simulink model "lab4_5"  (R2022b)
settings: Solver=ode5  StartTime=0.0  StopTime=10.0  FixedStep=0.1  RelTol=1e-3
values from neighbouring files (symbols this model uses):
  A0 = A0*1.5-A0*A0'*A0*0.5    [lab4.m]
  I_rotor = 0    [lab4.m]
  J = [I_x 0 0 ; 0 I_y 0; 0 0 I_z]    [lab4.m]
  k_rotor = [0, 0, 1]    [lab4.m]
  M = [M_x M_y M_z]    [lab4.m]
  omega = [omega_x, omega_y, omega_z]    [lab4.m]
  omega_rotor = 0    [lab4.m]
  q = 0.5.*OMEGA*q    [lab4.m]
libraries: vrlib x2
settings Model: Creator=paole  LastModifiedBy=a1pab
settings SolverCC: AlgebraicLoopSolver=TrustRegion
settings DebuggingCC: UnconnectedInputMsg=warning  UnconnectedOutputMsg=warning  UnconnectedLineMsg=warning  SFMachineParentedDataDiag=warning
settings ModelReferenceCC: EnableRefExpFcnMdlSchedulingChecks=on
settings RTWCC: DLArmComputeVersion=19.05

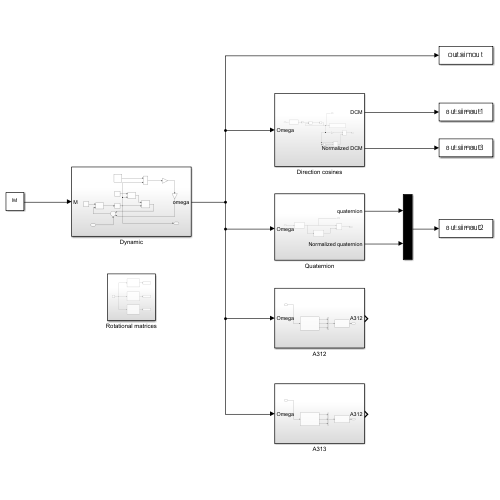
[thumbnail: Simulink's stored preview of the top-level diagram]
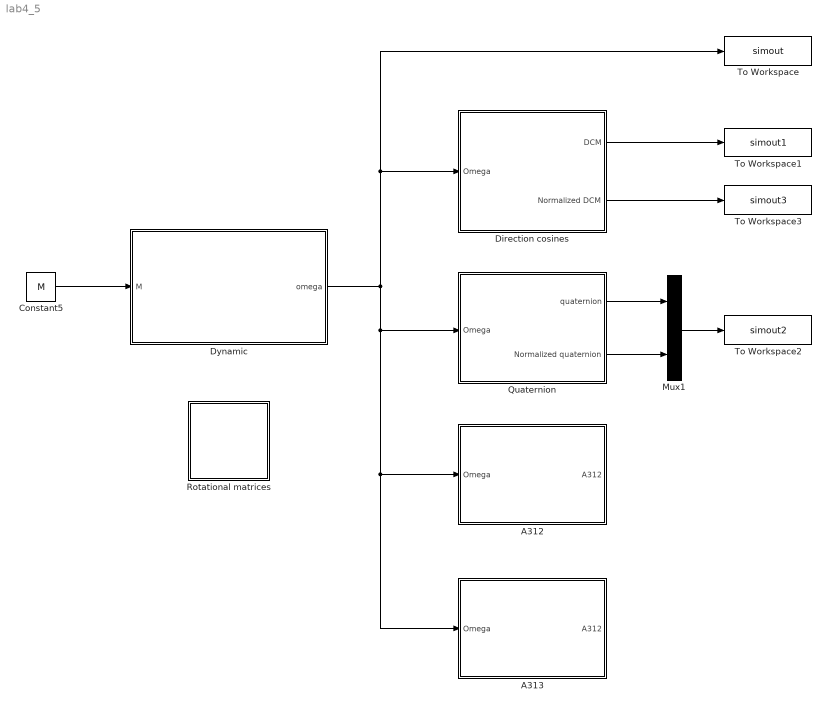
== system lab4_5 ==
  A312 : Subsystem
  A313 : Subsystem
  Constant5 : Constant  Value=M
  Direction cosines : Subsystem
  Dynamic : Subsystem
  Mux1 : Mux  Inputs=2
  Quaternion : Subsystem
  Rotational matrices : Subsystem
  To Workspace : ToWorkspace  VariableName=simout  SaveFormat=Timeseries  SampleTime=-1
  To Workspace1 : ToWorkspace  VariableName=simout1  SaveFormat=Timeseries  SampleTime=-1
  To Workspace2 : ToWorkspace  VariableName=simout2  SaveFormat=Timeseries  SampleTime=-1
  To Workspace3 : ToWorkspace  VariableName=simout3  SaveFormat=Timeseries  SampleTime=-1
  wires:
  Constant5/1 -> Dynamic/1(M)
  Dynamic/1(omega) -> Direction cosines/1(Omega), To Workspace/1, A313/1(Omega), A312/1(Omega), Quaternion/1(Omega)
  Direction cosines/1(DCM) -> To Workspace1/1
  Quaternion/2(Normalized quaternion) -> Mux1/2
  Quaternion/1(quaternion) -> Mux1/1
  Mux1/1 -> To Workspace2/1
  Direction cosines/2(Normalized DCM) -> To Workspace3/1

== system lab4_5/A312 ==
  Omega : Inport
  "Euler Angles 312 " : Subsystem
  Mux : Mux  Inputs=3
  Subsystem : Subsystem
  A312 : Outport
  wires:
  Subsystem/1(A312) -> A312/1
  "Euler Angles 312 "/3(Psi) -> Mux/3
  "Euler Angles 312 "/1(Phi) -> Mux/1
  "Euler Angles 312 "/2(Theta) -> Mux/2
  Mux/1 -> Subsystem/1("Phi, Theta, Psi")
  Omega/1 -> "Euler Angles 312 "/1(Omega)

== system lab4_5/A313 ==
  Omega : Inport
  "Euler Angles 313 " : Subsystem
  Mux : Mux  Inputs=3
  Subsystem : Subsystem
  A312 : Outport
  wires:
  Subsystem/1(A312) -> A312/1
  "Euler Angles 313 "/3(Psi) -> Mux/3
  "Euler Angles 313 "/1(Phi) -> Mux/1
  "Euler Angles 313 "/2(Theta) -> Mux/2
  Mux/1 -> Subsystem/1("Phi, Theta, Psi")
  Omega/1 -> "Euler Angles 313 "/1(Omega)

== system lab4_5/Direction cosines ==
  Omega : Inport
  Display1 : Display
  Gain : Gain  Gain=-1
  Gain1 : Gain  Gain=3/2
  Gain2 : Gain  Gain=1/2
  Integrator : Integrator  InitialCondition=A0
  Matrix Multiply : Product  Multiplication=Matrix(*)
  Matrix Multiply1 : Product  Inputs=3  Multiplication=Matrix(*)
  Subsystem : Subsystem
  Sum : Sum  Inputs=|+-
  Transpose : Math  Operator=transpose
  DCM : Outport
  Normalized DCM : Outport  Port=2
  wires:
  Matrix Multiply/1 -> Integrator/1
  Integrator/1 -> Matrix Multiply1/1, Transpose/1, Gain2/1, Gain1/1, DCM/1, Display1/1, Matrix Multiply/2
  Subsystem/1(W matrix) -> Gain/1
  Omega/1 -> Subsystem/1(Omega)
  Gain/1 -> Matrix Multiply/1
  Gain1/1 -> Sum/1
  Transpose/1 -> Matrix Multiply1/2
  Gain2/1 -> Matrix Multiply1/3
  Matrix Multiply1/1 -> Sum/2
  Sum/1 -> Normalized DCM/1

== system lab4_5/Dynamic ==
  M : Inport
  Constant : Constant  Value=k_rotor
  Constant2 : Constant  Value=J
  Constant3 : Constant  Value=inv(J)
  Cross Product : vrlib/Utilities/Cross Product
  Cross Product1 : vrlib/Utilities/Cross Product
  Gain : Gain  Gain=omega_rotor
  I_r : Gain  Gain=I_rotor
  Integrator3 : Integrator  InitialCondition=omega
  Matrix Multiply : Product  Multiplication=Matrix(*)
  Matrix Multiply1 : Product  Multiplication=Matrix(*)
  Sum6 : Sum  Inputs=|+++
  omega : Outport
  wires:
  Integrator3/1 -> omega/1, Cross Product/2, Cross Product1/2, Matrix Multiply1/2  "omega"
  Sum6/1 -> Matrix Multiply/2  "J*omega'"
  Constant3/1 -> Matrix Multiply/1
  Matrix Multiply/1 -> Integrator3/1  "omega'"
  Matrix Multiply1/1 -> Cross Product/1  "Jw"
  Constant2/1 -> Matrix Multiply1/1
  Cross Product/1 -> Sum6/1  "Jw^w"
  Constant/1 -> Cross Product1/1
  Cross Product1/1 -> I_r/1  "k*omega"
  M/1 -> Sum6/3
  I_r/1 -> Gain/1  "k*omega*I_r"
  Gain/1 -> Sum6/2  "k*Wr*W*I_r"

== system lab4_5/Quaternion ==
  Omega : Inport
  Divide : Product  Inputs=*/
  Quaternion : Subsystem
  Subsystem : Subsystem
  quaternion : Outport
  Normalized quaternion : Outport  Port=2
  wires:
  Quaternion/1(Quaternion) -> quaternion/1, Divide/1, Subsystem/1(Quaternion)
  Omega/1 -> Quaternion/1(Omega)
  Subsystem/1(Norm) -> Divide/2
  Divide/1 -> Normalized quaternion/1

== system lab4_5/Rotational matrices ==
  Constant : Constant
  Display : Display
  Display1 : Display
  Display2 : Display
  Rotation around first axis : Subsystem
  Rotation around second axis : Subsystem
  Rotation around third axis : Subsystem
  wires:
  Rotation around third axis/1(A3) -> Display2/1
  Rotation around first axis/1(A1) -> Display1/1
  Rotation around second axis/1(A2) -> Display/1
  Constant/1 -> Rotation around third axis/1(angle), Rotation around first axis/1(angle), Rotation around second axis/1(angle)

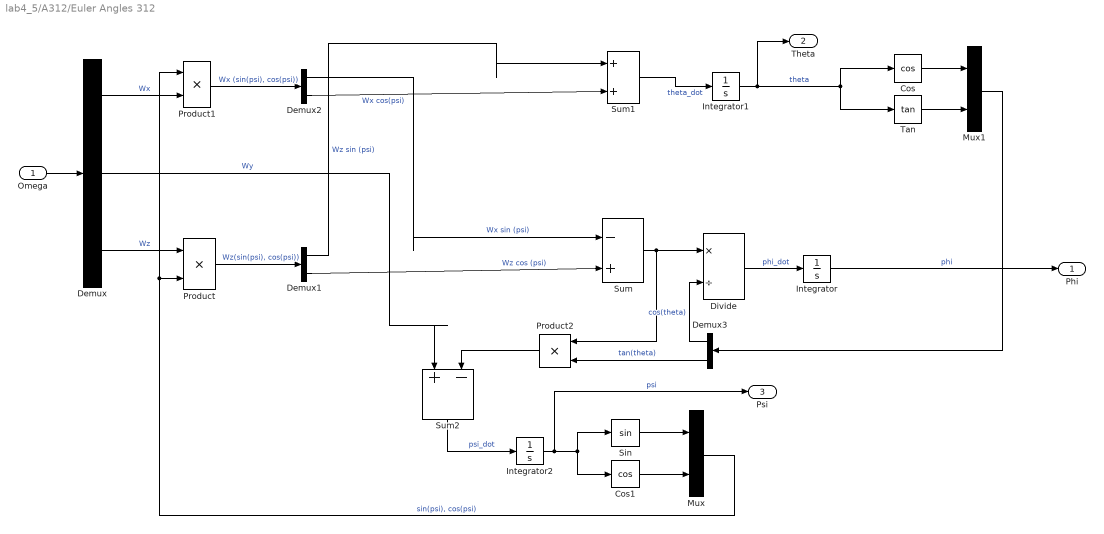
== system lab4_5/A312/Euler Angles 312  ==
  Omega : Inport
  Cos : Trigonometry  Operator=cos
  Cos1 : Trigonometry  Operator=cos
  Demux : Demux  Outputs=3
  Demux1 : Demux  Outputs=2
  Demux2 : Demux  Outputs=2
  Demux3 : Demux  Outputs=2
  Divide : Product  Inputs=*/
  Integrator : Integrator
  Integrator1 : Integrator
  Integrator2 : Integrator
  Mux : Mux  Inputs=2
  Mux1 : Mux  Inputs=2
  Product : Product
  Product1 : Product
  Product2 : Product
  Sin : Trigonometry
  Sum : Sum  Inputs=|-+
  Sum1 : Sum  Inputs=|++
  Sum2 : Sum  Inputs=|+-
  Tan : Trigonometry  Operator=tan
  Phi : Outport
  Theta : Outport  Port=2
  Psi : Outport  Port=3
  wires:
  Omega/1 -> Demux/1
  Demux/3 -> Product/1  "Wz"
  Demux/2 -> Sum2/1  "Wy"
  Demux/1 -> Product1/2  "Wx"
  Sum/1 -> Divide/1, Product2/1
  Divide/1 -> Integrator/1  "phi_dot"
  Integrator/1 -> Phi/1  "phi"
  Demux2/1 -> Sum/1  "Wx sin (psi)"
  Demux1/2 -> Sum/2  "Wz cos (psi)"
  Demux1/1 -> Sum1/1  "Wz sin (psi)"
  Demux2/2 -> Sum1/2  "Wx cos(psi)"
  Sum1/1 -> Integrator1/1  "theta_dot"
  Integrator1/1 -> Theta/1, Tan/1, Cos/1  "theta"
  Mux1/1 -> Demux3/1
  Demux3/1 -> Divide/2  "cos(theta)"
  Demux3/2 -> Product2/2  "tan(theta)"
  Cos/1 -> Mux1/1
  Tan/1 -> Mux1/2
  Product2/1 -> Sum2/2
  Sum2/1 -> Integrator2/1  "psi_dot"
  Integrator2/1 -> Psi/1, Cos1/1, Sin/1  "psi"
  Sin/1 -> Mux/1
  Cos1/1 -> Mux/2
  Mux/1 -> Product1/1, Product/2  "sin(psi), cos(psi)"
  Product/1 -> Demux1/1  "Wz(sin(psi), cos(psi))"
  Product1/1 -> Demux2/1  "Wx (sin(psi), cos(psi))"

== system lab4_5/A312/Subsystem ==
  "Phi, Theta, Psi" : Inport
  Cos : Trigonometry  Operator=cos
  Display : Display
  First vector row : Subsystem
  Matrix Concatenate : Concatenate  NumInputs=3  Mode=Multidimensional array
  Second vector row : Subsystem
  Sin : Trigonometry
  Third vector Row : Subsystem
  A312 : Outport
  wires:
  "Phi, Theta, Psi"/1 -> Cos/1, Sin/1
  Cos/1 -> Second vector row/1(In1), Third vector Row/1(In1), First vector row/1(In1)
  Sin/1 -> Second vector row/2(In2), First vector row/2(In2), Third vector Row/2(In2)
  First vector row/1(Output) -> Matrix Concatenate/1
  Second vector row/1(Output) -> Matrix Concatenate/2
  Third vector Row/1(Output) -> Matrix Concatenate/3
  Matrix Concatenate/1 -> A312/1, Display/1

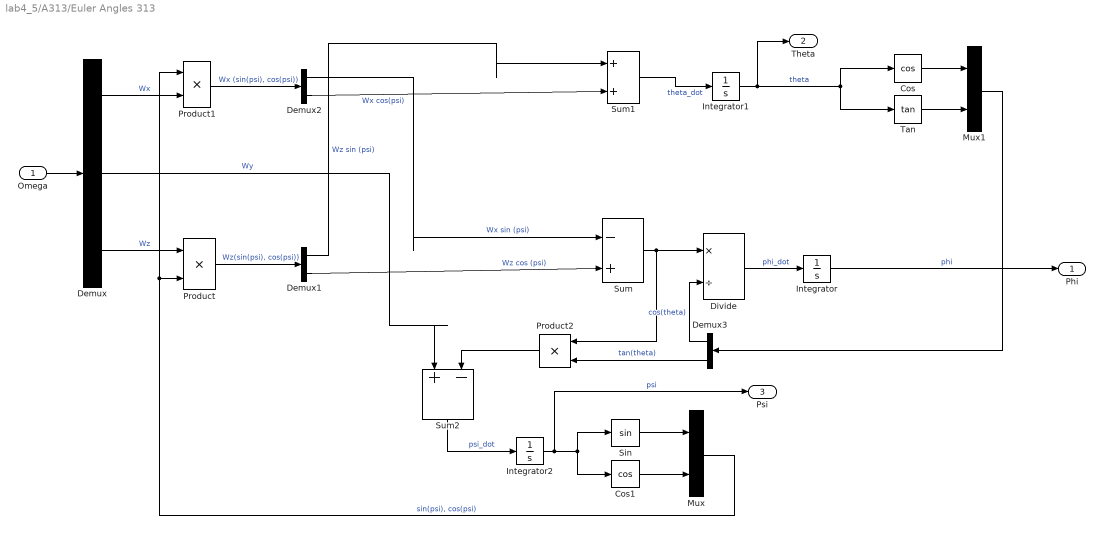
== system lab4_5/A313/Euler Angles 313  ==
  Omega : Inport
  Cos : Trigonometry  Operator=cos
  Cos1 : Trigonometry  Operator=cos
  Demux : Demux  Outputs=3
  Demux1 : Demux  Outputs=2
  Demux2 : Demux  Outputs=2
  Demux3 : Demux  Outputs=2
  Divide : Product  Inputs=*/
  Integrator : Integrator
  Integrator1 : Integrator
  Integrator2 : Integrator
  Mux : Mux  Inputs=2
  Mux1 : Mux  Inputs=2
  Product : Product
  Product1 : Product
  Product2 : Product
  Sin : Trigonometry
  Sum : Sum  Inputs=|-+
  Sum1 : Sum  Inputs=|++
  Sum2 : Sum  Inputs=|+-
  Tan : Trigonometry  Operator=tan
  Phi : Outport
  Theta : Outport  Port=2
  Psi : Outport  Port=3
  wires:
  Omega/1 -> Demux/1
  Demux/3 -> Product/1  "Wz"
  Demux/2 -> Sum2/1  "Wy"
  Demux/1 -> Product1/2  "Wx"
  Sum/1 -> Divide/1, Product2/1
  Divide/1 -> Integrator/1  "phi_dot"
  Integrator/1 -> Phi/1  "phi"
  Demux2/1 -> Sum/1  "Wx sin (psi)"
  Demux1/2 -> Sum/2  "Wz cos (psi)"
  Demux1/1 -> Sum1/1  "Wz sin (psi)"
  Demux2/2 -> Sum1/2  "Wx cos(psi)"
  Sum1/1 -> Integrator1/1  "theta_dot"
  Integrator1/1 -> Theta/1, Tan/1, Cos/1  "theta"
  Mux1/1 -> Demux3/1
  Demux3/1 -> Divide/2  "cos(theta)"
  Demux3/2 -> Product2/2  "tan(theta)"
  Cos/1 -> Mux1/1
  Tan/1 -> Mux1/2
  Product2/1 -> Sum2/2
  Sum2/1 -> Integrator2/1  "psi_dot"
  Integrator2/1 -> Psi/1, Cos1/1, Sin/1  "psi"
  Sin/1 -> Mux/1
  Cos1/1 -> Mux/2
  Mux/1 -> Product1/1, Product/2  "sin(psi), cos(psi)"
  Product/1 -> Demux1/1  "Wz(sin(psi), cos(psi))"
  Product1/1 -> Demux2/1  "Wx (sin(psi), cos(psi))"

== system lab4_5/A313/Subsystem ==
  "Phi, Theta, Psi" : Inport
  Cos : Trigonometry  Operator=cos
  Display : Display
  First vector row : Subsystem
  Matrix Concatenate : Concatenate  NumInputs=3  Mode=Multidimensional array
  Second vector row : Subsystem
  Sin : Trigonometry
  Third vector Row : Subsystem
  A312 : Outport
  wires:
  "Phi, Theta, Psi"/1 -> Cos/1, Sin/1
  Cos/1 -> Second vector row/1(In1), Third vector Row/1(In1), First vector row/1(In1)
  Sin/1 -> Second vector row/2(In2), First vector row/2(In2), Third vector Row/2(In2)
  First vector row/1(Output) -> Matrix Concatenate/1
  Second vector row/1(Output) -> Matrix Concatenate/2
  Third vector Row/1(Output) -> Matrix Concatenate/3
  Matrix Concatenate/1 -> A312/1, Display/1

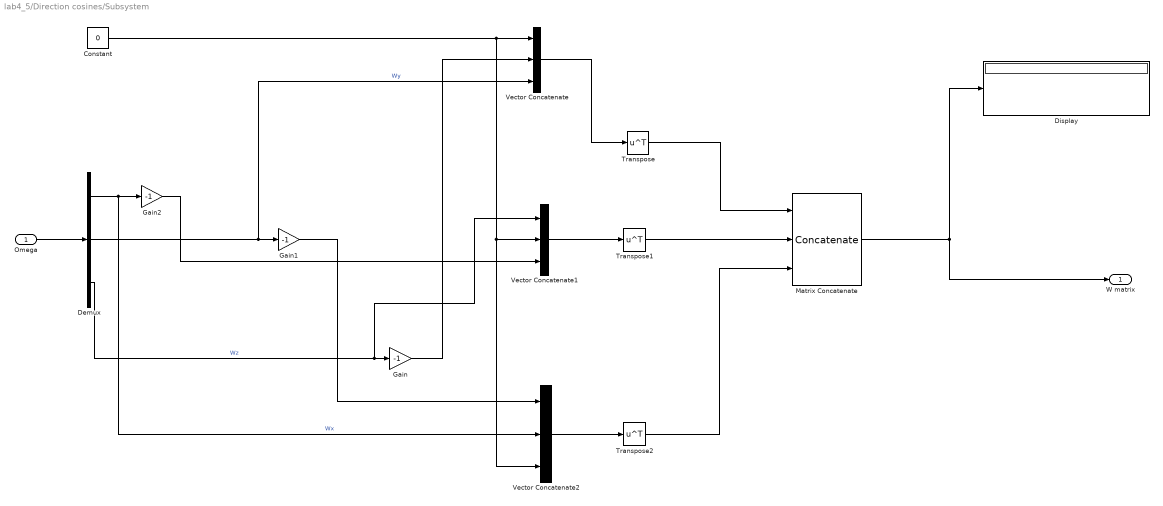
== system lab4_5/Direction cosines/Subsystem ==
  Omega : Inport
  Constant : Constant  Value=0
  Demux : Demux  Outputs=3
  Display : Display
  Gain : Gain  Gain=-1
  Gain1 : Gain  Gain=-1
  Gain2 : Gain  Gain=-1
  Matrix Concatenate : Concatenate  NumInputs=3  Mode=Multidimensional array
  Transpose : Math  Operator=transpose
  Transpose1 : Math  Operator=transpose
  Transpose2 : Math  Operator=transpose
  Vector Concatenate : Concatenate  NumInputs=3
  Vector Concatenate1 : Concatenate  NumInputs=3
  Vector Concatenate2 : Concatenate  NumInputs=3
  W matrix : Outport
  wires:
  Omega/1 -> Demux/1
  Demux/3 -> Vector Concatenate1/1, Gain/1  "Wz"
  Demux/1 -> Vector Concatenate2/2, Gain2/1  "Wx"
  Demux/2 -> Gain1/1, Vector Concatenate/3  "Wy"
  Constant/1 -> Vector Concatenate2/3, Vector Concatenate1/2, Vector Concatenate/1
  Gain/1 -> Vector Concatenate/2
  Vector Concatenate/1 -> Transpose/1
  Gain2/1 -> Vector Concatenate1/3
  Gain1/1 -> Vector Concatenate2/1
  Vector Concatenate1/1 -> Transpose1/1
  Vector Concatenate2/1 -> Transpose2/1
  Matrix Concatenate/1 -> W matrix/1, Display/1
  Transpose2/1 -> Matrix Concatenate/3
  Transpose1/1 -> Matrix Concatenate/2
  Transpose/1 -> Matrix Concatenate/1

== system lab4_5/Quaternion/Quaternion ==
  Omega : Inport
  Display : Display
  Gain : Gain  Gain=1/2
  Integrator : Integrator  InitialCondition=q
  Matrix Multiply : Product  Multiplication=Matrix(*)
  Quaternions : Subsystem
  Quaternion : Outport
  wires:
  Gain/1 -> Matrix Multiply/1
  Quaternions/1(OMEGA_matrix) -> Gain/1
  Matrix Multiply/1 -> Integrator/1
  Integrator/1 -> Display/1, Quaternion/1, Matrix Multiply/2
  Omega/1 -> Quaternions/1(Omega)

== system lab4_5/Quaternion/Subsystem ==
  Quaternion : Inport
  Demux : Demux
  Product{,1..3} (4 alike) : Product
  Sqrt : Sqrt
  Sum : Sum  Inputs=|++++
  Norm : Outport
  wires:
  Quaternion/1 -> Demux/1
  Demux/1 -> Product/2, Product/1
  Demux/2 -> Product1/2, Product1/1
  Demux/3 -> Product2/2, Product2/1
  Demux/4 -> Product3/2, Product3/1
  Product/1 -> Sum/1
  Product2/1 -> Sum/3
  Product1/1 -> Sum/2
  Product3/1 -> Sum/4
  Sum/1 -> Sqrt/1
  Sqrt/1 -> Norm/1

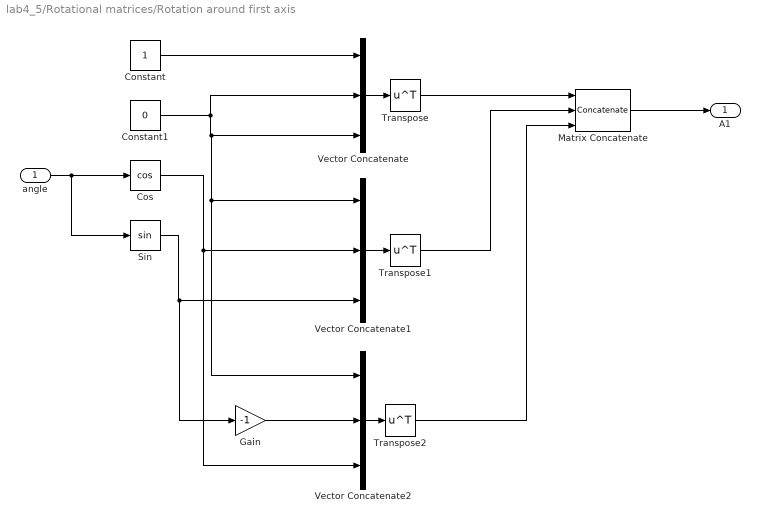
== system lab4_5/Rotational matrices/Rotation around first axis ==
  angle : Inport
  Constant : Constant
  Constant1 : Constant  Value=0
  Cos : Trigonometry  Operator=cos
  Gain : Gain  Gain=-1
  Matrix Concatenate : Concatenate  NumInputs=3  Mode=Multidimensional array
  Sin : Trigonometry
  Transpose : Math  Operator=transpose
  Transpose1 : Math  Operator=transpose
  Transpose2 : Math  Operator=transpose
  Vector Concatenate : Concatenate  NumInputs=3
  Vector Concatenate1 : Concatenate  NumInputs=3
  Vector Concatenate2 : Concatenate  NumInputs=3
  A1 : Outport
  wires:
  angle/1 -> Sin/1, Cos/1
  Sin/1 -> Gain/1, Vector Concatenate1/3
  Constant/1 -> Vector Concatenate/1
  Constant1/1 -> Vector Concatenate1/1, Vector Concatenate2/1, Vector Concatenate/3, Vector Concatenate/2
  Vector Concatenate/1 -> Transpose/1
  Transpose/1 -> Matrix Concatenate/1
  Cos/1 -> Vector Concatenate2/3, Vector Concatenate1/2
  Vector Concatenate1/1 -> Transpose1/1
  Transpose1/1 -> Matrix Concatenate/2
  Gain/1 -> Vector Concatenate2/2
  Vector Concatenate2/1 -> Transpose2/1
  Transpose2/1 -> Matrix Concatenate/3
  Matrix Concatenate/1 -> A1/1

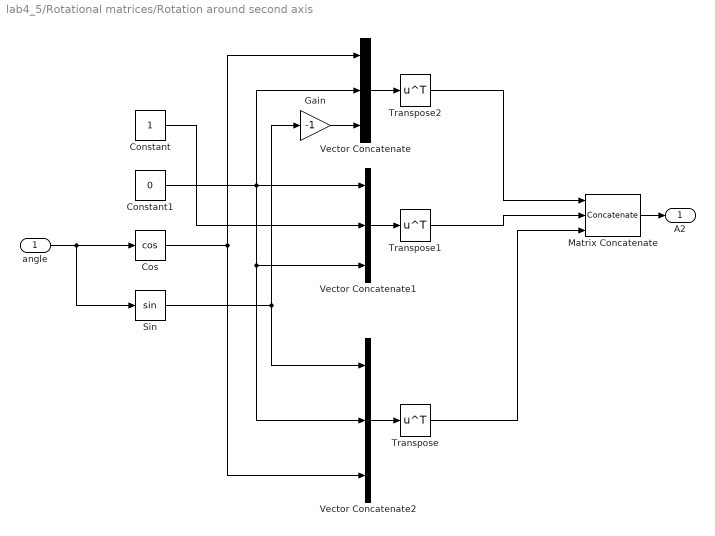
== system lab4_5/Rotational matrices/Rotation around second axis ==
  angle : Inport
  Constant : Constant
  Constant1 : Constant  Value=0
  Cos : Trigonometry  Operator=cos
  Gain : Gain  Gain=-1
  Matrix Concatenate : Concatenate  NumInputs=3  Mode=Multidimensional array
  Sin : Trigonometry
  Transpose : Math  Operator=transpose
  Transpose1 : Math  Operator=transpose
  Transpose2 : Math  Operator=transpose
  Vector Concatenate : Concatenate  NumInputs=3
  Vector Concatenate1 : Concatenate  NumInputs=3
  Vector Concatenate2 : Concatenate  NumInputs=3
  A2 : Outport
  wires:
  angle/1 -> Sin/1, Cos/1
  Constant1/1 -> Vector Concatenate1/1, Vector Concatenate2/2, Vector Concatenate1/3, Vector Concatenate/2
  Constant/1 -> Vector Concatenate1/2
  Cos/1 -> Vector Concatenate2/3, Vector Concatenate/1
  Sin/1 -> Vector Concatenate2/1, Gain/1
  Gain/1 -> Vector Concatenate/3
  Vector Concatenate2/1 -> Transpose/1
  Vector Concatenate1/1 -> Transpose1/1
  Vector Concatenate/1 -> Transpose2/1
  Transpose2/1 -> Matrix Concatenate/1
  Transpose1/1 -> Matrix Concatenate/2
  Transpose/1 -> Matrix Concatenate/3
  Matrix Concatenate/1 -> A2/1

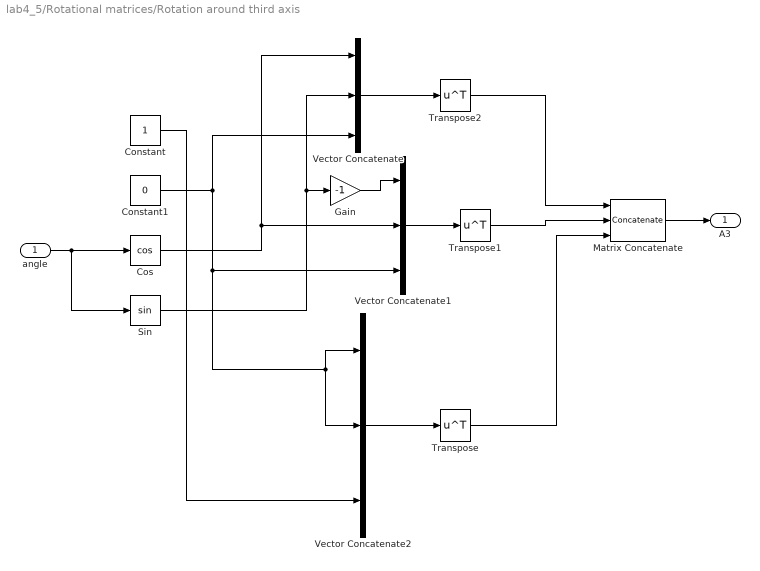
== system lab4_5/Rotational matrices/Rotation around third axis ==
  angle : Inport
  Constant : Constant
  Constant1 : Constant  Value=0
  Cos : Trigonometry  Operator=cos
  Gain : Gain  Gain=-1
  Matrix Concatenate : Concatenate  NumInputs=3  Mode=Multidimensional array
  Sin : Trigonometry
  Transpose : Math  Operator=transpose
  Transpose1 : Math  Operator=transpose
  Transpose2 : Math  Operator=transpose
  Vector Concatenate : Concatenate  NumInputs=3
  Vector Concatenate1 : Concatenate  NumInputs=3
  Vector Concatenate2 : Concatenate  NumInputs=3
  A3 : Outport
  wires:
  angle/1 -> Sin/1, Cos/1
  Sin/1 -> Vector Concatenate/2, Gain/1
  Cos/1 -> Vector Concatenate/1, Vector Concatenate1/2
  Constant1/1 -> Vector Concatenate2/2, Vector Concatenate2/1, Vector Concatenate1/3, Vector Concatenate/3
  Gain/1 -> Vector Concatenate1/1
  Constant/1 -> Vector Concatenate2/3
  Vector Concatenate2/1 -> Transpose/1
  Vector Concatenate1/1 -> Transpose1/1
  Vector Concatenate/1 -> Transpose2/1
  Transpose2/1 -> Matrix Concatenate/1
  Transpose1/1 -> Matrix Concatenate/2
  Transpose/1 -> Matrix Concatenate/3
  Matrix Concatenate/1 -> A3/1

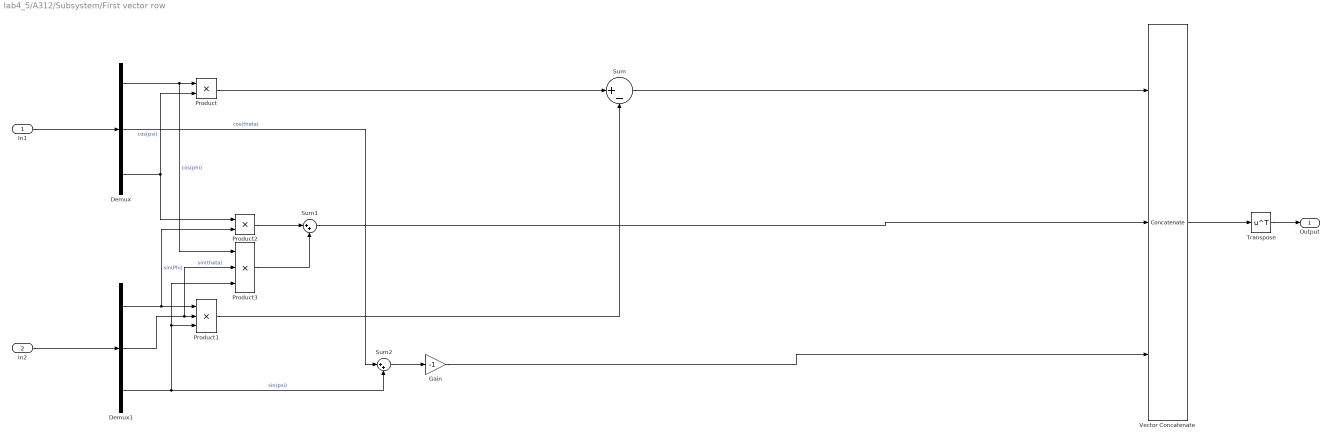
== system lab4_5/A312/Subsystem/First vector row ==
  In1 : Inport
  In2 : Inport  Port=2
  Demux : Demux  Outputs=3
  Demux1 : Demux  Outputs=3
  Gain : Gain  Gain=-1
  Product : Product
  Product1 : Product  Inputs=3
  Product2 : Product
  Product3 : Product  Inputs=3
  Sum : Sum  Inputs=|+-
  Sum1 : Sum  Inputs=|++
  Sum2 : Sum  Inputs=|++
  Transpose : Math  Operator=transpose
  Vector Concatenate : Concatenate  NumInputs=3
  Output : Outport
  wires:
  In2/1 -> Demux1/1
  In1/1 -> Demux/1
  Demux1/1 -> Product1/1, Product2/2  "sin(Phi)"
  Demux/2 -> Sum2/1  "cos(theta)"
  Demux1/2 -> Product3/2, Product1/2  "sin(theta)"
  Demux1/3 -> Sum2/2, Product3/3, Product1/3  "sin(psi)"
  Demux/1 -> Product3/1, Product/1  "cos(phi)"
  Demux/3 -> Product2/1, Product/2  "cos(psi)"
  Product1/1 -> Sum/2
  Product/1 -> Sum/1
  Sum/1 -> Vector Concatenate/1
  Product2/1 -> Sum1/1
  Product3/1 -> Sum1/2
  Sum2/1 -> Gain/1
  Sum1/1 -> Vector Concatenate/2
  Gain/1 -> Vector Concatenate/3
  Vector Concatenate/1 -> Transpose/1
  Transpose/1 -> Output/1

== system lab4_5/A312/Subsystem/Second vector row ==
  In1 : Inport
  In2 : Inport  Port=2
  Demux : Demux  Outputs=3
  Demux1 : Demux  Outputs=3
  Gain : Gain  Gain=-1
  Product : Product
  Product1 : Product
  Scope : Scope
  Scope1 : Scope
  Transpose : Math  Operator=transpose
  Vector Concatenate : Concatenate  NumInputs=3
  Output : Outport
  wires:
  Demux1/1 -> Product/2  "sin(Phi)"
  Demux/2 -> Product1/2, Product/1  "cos(theta)"
  Demux1/2 -> Vector Concatenate/3  "sin(theta)"
  Demux1/3 -> Scope1/1  "sin(psi)"
  Demux/1 -> Product1/1  "cos(phi)"
  Demux/3 -> Scope/1  "cos(psi)"
  In2/1 -> Demux1/1
  In1/1 -> Demux/1
  Product/1 -> Gain/1
  Gain/1 -> Vector Concatenate/1
  Product1/1 -> Vector Concatenate/2
  Vector Concatenate/1 -> Transpose/1
  Transpose/1 -> Output/1

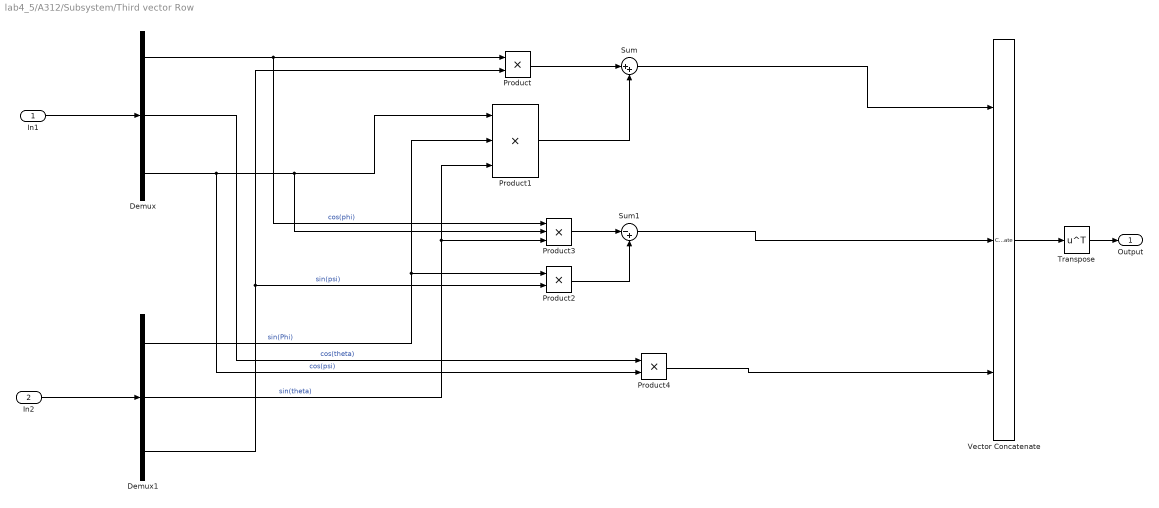
== system lab4_5/A312/Subsystem/Third vector Row ==
  In1 : Inport
  In2 : Inport  Port=2
  Demux : Demux  Outputs=3
  Demux1 : Demux  Outputs=3
  Product : Product
  Product1 : Product  Inputs=3
  Product2 : Product
  Product3 : Product  Inputs=3
  Product4 : Product
  Sum : Sum  Inputs=|++
  Sum1 : Sum  Inputs=|-+
  Transpose : Math  Operator=transpose
  Vector Concatenate : Concatenate  NumInputs=3
  Output : Outport
  wires:
  In2/1 -> Demux1/1
  In1/1 -> Demux/1
  Demux1/1 -> Product2/1, Product1/2  "sin(Phi)"
  Demux/2 -> Product4/1  "cos(theta)"
  Demux1/2 -> Product1/3, Product3/3  "sin(theta)"
  Demux1/3 -> Product2/2, Product/2  "sin(psi)"
  Demux/1 -> Product3/1, Product/1  "cos(phi)"
  Demux/3 -> Product4/2, Product3/2, Product1/1  "cos(psi)"
  Product/1 -> Sum/1
  Product1/1 -> Sum/2
  Sum/1 -> Vector Concatenate/1
  Product2/1 -> Sum1/2
  Product3/1 -> Sum1/1
  Sum1/1 -> Vector Concatenate/2
  Product4/1 -> Vector Concatenate/3
  Vector Concatenate/1 -> Transpose/1
  Transpose/1 -> Output/1

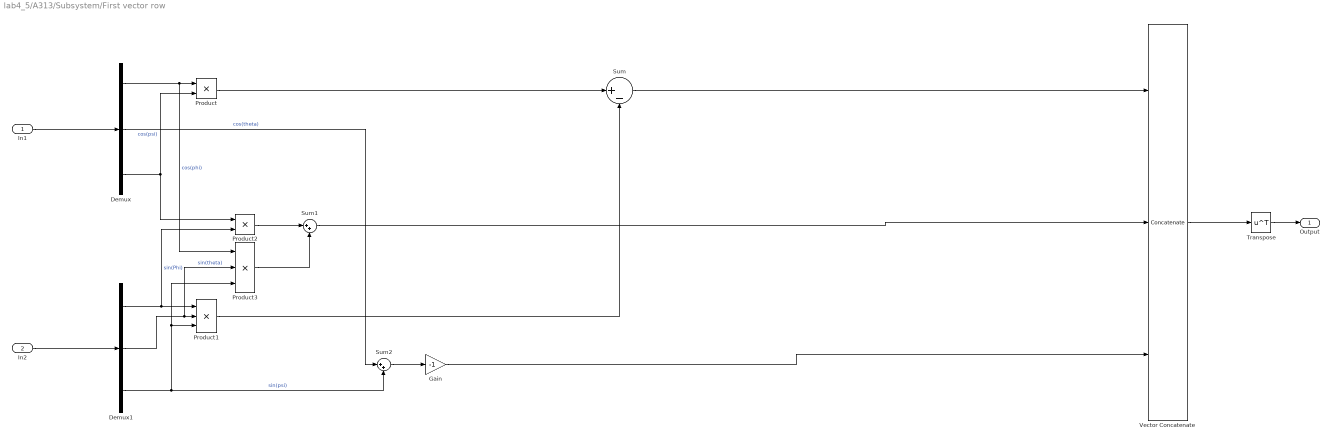
== system lab4_5/A313/Subsystem/First vector row ==
  In1 : Inport
  In2 : Inport  Port=2
  Demux : Demux  Outputs=3
  Demux1 : Demux  Outputs=3
  Gain : Gain  Gain=-1
  Product : Product
  Product1 : Product  Inputs=3
  Product2 : Product
  Product3 : Product  Inputs=3
  Sum : Sum  Inputs=|+-
  Sum1 : Sum  Inputs=|++
  Sum2 : Sum  Inputs=|++
  Transpose : Math  Operator=transpose
  Vector Concatenate : Concatenate  NumInputs=3
  Output : Outport
  wires:
  In2/1 -> Demux1/1
  In1/1 -> Demux/1
  Demux1/1 -> Product1/1, Product2/2  "sin(Phi)"
  Demux/2 -> Sum2/1  "cos(theta)"
  Demux1/2 -> Product3/2, Product1/2  "sin(theta)"
  Demux1/3 -> Sum2/2, Product3/3, Product1/3  "sin(psi)"
  Demux/1 -> Product3/1, Product/1  "cos(phi)"
  Demux/3 -> Product2/1, Product/2  "cos(psi)"
  Product1/1 -> Sum/2
  Product/1 -> Sum/1
  Sum/1 -> Vector Concatenate/1
  Product2/1 -> Sum1/1
  Product3/1 -> Sum1/2
  Sum2/1 -> Gain/1
  Sum1/1 -> Vector Concatenate/2
  Gain/1 -> Vector Concatenate/3
  Vector Concatenate/1 -> Transpose/1
  Transpose/1 -> Output/1

== system lab4_5/A313/Subsystem/Second vector row ==
  In1 : Inport
  In2 : Inport  Port=2
  Demux : Demux  Outputs=3
  Demux1 : Demux  Outputs=3
  Gain : Gain  Gain=-1
  Product : Product
  Product1 : Product
  Scope : Scope
  Scope1 : Scope
  Transpose : Math  Operator=transpose
  Vector Concatenate : Concatenate  NumInputs=3
  Output : Outport
  wires:
  Demux1/1 -> Product/2  "sin(Phi)"
  Demux/2 -> Product1/2, Product/1  "cos(theta)"
  Demux1/2 -> Vector Concatenate/3  "sin(theta)"
  Demux1/3 -> Scope1/1  "sin(psi)"
  Demux/1 -> Product1/1  "cos(phi)"
  Demux/3 -> Scope/1  "cos(psi)"
  In2/1 -> Demux1/1
  In1/1 -> Demux/1
  Product/1 -> Gain/1
  Gain/1 -> Vector Concatenate/1
  Product1/1 -> Vector Concatenate/2
  Vector Concatenate/1 -> Transpose/1
  Transpose/1 -> Output/1

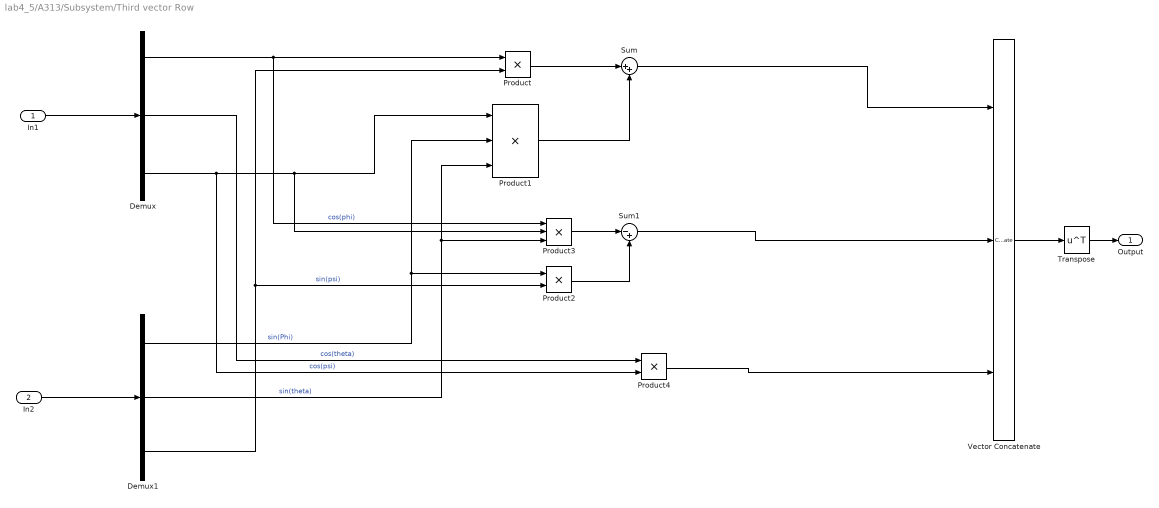
== system lab4_5/A313/Subsystem/Third vector Row ==
  In1 : Inport
  In2 : Inport  Port=2
  Demux : Demux  Outputs=3
  Demux1 : Demux  Outputs=3
  Product : Product
  Product1 : Product  Inputs=3
  Product2 : Product
  Product3 : Product  Inputs=3
  Product4 : Product
  Sum : Sum  Inputs=|++
  Sum1 : Sum  Inputs=|-+
  Transpose : Math  Operator=transpose
  Vector Concatenate : Concatenate  NumInputs=3
  Output : Outport
  wires:
  In2/1 -> Demux1/1
  In1/1 -> Demux/1
  Demux1/1 -> Product2/1, Product1/2  "sin(Phi)"
  Demux/2 -> Product4/1  "cos(theta)"
  Demux1/2 -> Product1/3, Product3/3  "sin(theta)"
  Demux1/3 -> Product2/2, Product/2  "sin(psi)"
  Demux/1 -> Product3/1, Product/1  "cos(phi)"
  Demux/3 -> Product4/2, Product3/2, Product1/1  "cos(psi)"
  Product/1 -> Sum/1
  Product1/1 -> Sum/2
  Sum/1 -> Vector Concatenate/1
  Product2/1 -> Sum1/2
  Product3/1 -> Sum1/1
  Sum1/1 -> Vector Concatenate/2
  Product4/1 -> Vector Concatenate/3
  Vector Concatenate/1 -> Transpose/1
  Transpose/1 -> Output/1

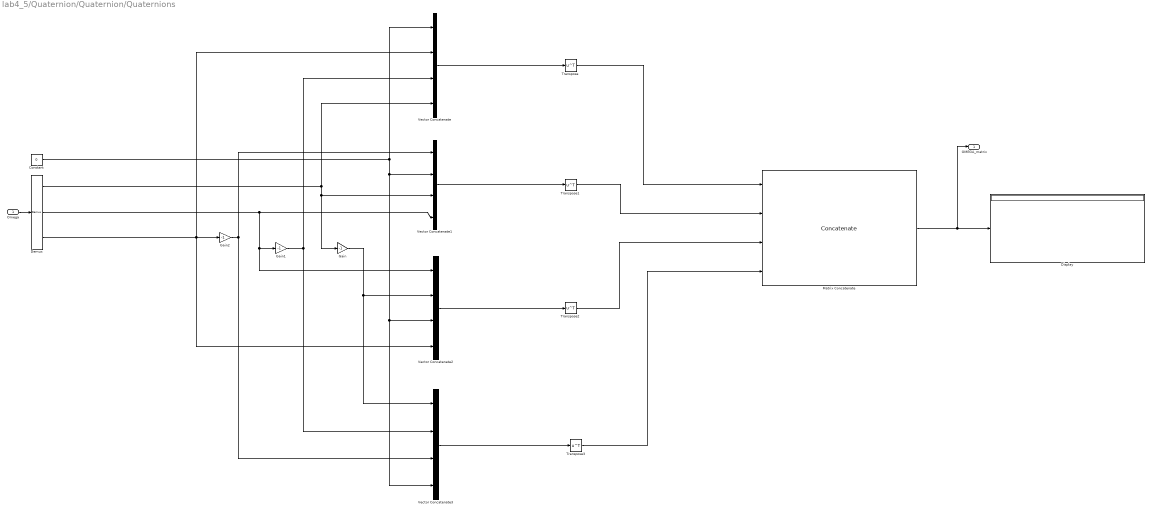
== system lab4_5/Quaternion/Quaternion/Quaternions ==
  Omega : Inport
  Constant : Constant  Value=0
  Demux : Demux  Outputs=3
  Display : Display
  Gain : Gain  Gain=-1
  Gain1 : Gain  Gain=-1
  Gain2 : Gain  Gain=-1
  Matrix Concatenate : Concatenate  NumInputs=4  Mode=Multidimensional array
  Transpose{,1..3} (4 alike) : Math  Operator=transpose
  Vector Concatenate{,1..3} (4 alike) : Concatenate  NumInputs=4
  OMEGA_matrix : Outport
  wires:
  Omega/1 -> Demux/1
  Demux/1 -> Vector Concatenate1/3, Gain/1, Vector Concatenate/4
  Demux/2 -> Vector Concatenate2/1, Gain1/1, Vector Concatenate1/4
  Demux/3 -> Vector Concatenate2/4, Vector Concatenate/2, Gain2/1
  Constant/1 -> Vector Concatenate/1, Vector Concatenate2/3, Vector Concatenate3/4, Vector Concatenate1/2
  Vector Concatenate2/1 -> Transpose2/1
  Gain/1 -> Vector Concatenate3/1, Vector Concatenate2/2
  Gain1/1 -> Vector Concatenate3/2, Vector Concatenate/3
  Gain2/1 -> Vector Concatenate3/3, Vector Concatenate1/1
  Vector Concatenate/1 -> Transpose/1
  Vector Concatenate1/1 -> Transpose1/1
  Vector Concatenate3/1 -> Transpose3/1
  Transpose/1 -> Matrix Concatenate/1
  Transpose1/1 -> Matrix Concatenate/2
  Transpose2/1 -> Matrix Concatenate/3
  Transpose3/1 -> Matrix Concatenate/4
  Matrix Concatenate/1 -> OMEGA_matrix/1, Display/1
